simulink model "srf_pll"  (R2023a)
settings: configuration reference "Configuration" (kept outside this file)
values from neighbouring files (symbols this model uses):
  tsample = 0.0002    [dictionary_srf_pll.sldd]
settings Model: DataDictionary=dictionary_srf_pll.sldd  Creator=ASUSTUF  LastModifiedBy=ASUSTUF
settings ConfigSetRef: SourceName=Configuration

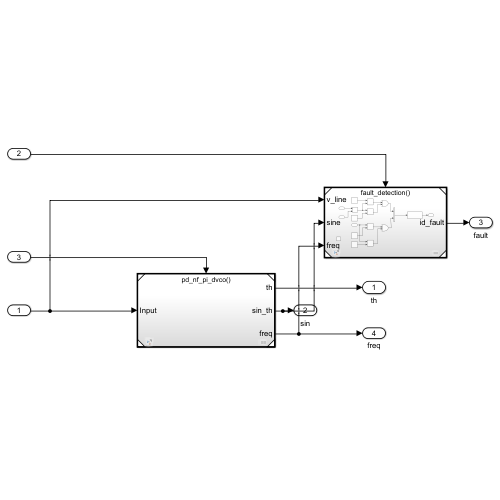
[thumbnail: Simulink's stored preview of the top-level diagram]
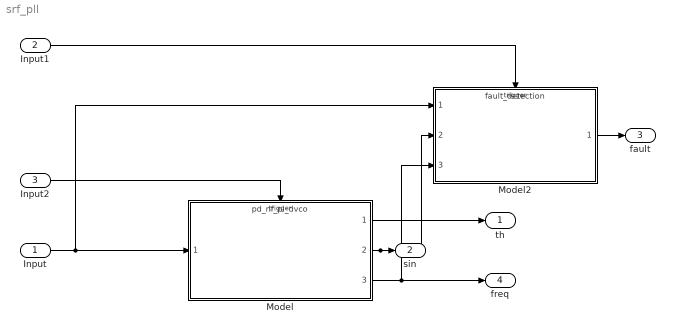
== system srf_pll ==
  Input : Inport
  Input1 : Inport  Port=2  SampleTime=tsample  OutputFunctionCall=on
  Input2 : Inport  Port=3  SampleTime=tsample  OutputFunctionCall=on
  Model : ModelReference  ModelNameDialog=pd_nf_pi_dvco.slx  SimulationMode=Normal  ModelReferenceVersion=1.31  TriggerPortName=Trigger  TriggerPortTriggerType=function-call  TriggerPortStatesWhenEnabling=held
  Model2 : ModelReference  ModelNameDialog=fault_detection.slx  SimulationMode=Normal  ModelReferenceVersion=1.12  TriggerPortName=Trigger  TriggerPortTriggerType=function-call  TriggerPortStatesWhenEnabling=held
  th : Outport
  sin : Outport  Port=2
  fault : Outport  Port=3
  freq : Outport  Port=4
  wires:
  Input1/1 -> Model2/Trigger
  Input/1 -> Model2/1, Model/1
  Input2/1 -> Model/Trigger
  Model2/1 -> fault/1
  Model/2 -> Model2/2, sin/1
  Model/1 -> th/1
  Model/3 -> Model2/3, freq/1
